simulink model "brain"  (Simulink 7.5)
settings: Solver=FixedStepDiscrete  StartTime=0.0  StopTime=inf  FixedStep=0.2  RelTol=1e-3
values from neighbouring files (symbols this model uses):
  Buoy1_Hue = 0.4    [brainconstants.m]    (also in brainconstants_David.m = 30)
  Buoy1_Saturation = 1.0    (= 1)    [brainconstants.m]    (also in brainconstants_David.m)
  Buoy1_Value = 0.45    [brainconstants.m]    (also in brainconstants_David.m)
  Buoy2_Hue = 0.0    (= 0)    [brainconstants.m]    (also in brainconstants_David.m = 80)
  Buoy2_Saturation = 1.0    (= 1)    [brainconstants.m]    (also in brainconstants_David.m)
  Buoy2_Value = 0.75    [brainconstants.m]    (also in brainconstants_David.m)
  Buoy_Max_Eccentricity = 0.7    [brainconstants.m]    (also in brainconstants_David.m = 1.2)
  Buoy_Max_Extent = 0.9    [brainconstants.m]    (also in brainconstants_David.m)
  Buoy_Min_Eccentricity = 0    [brainconstants.m]    (also in brainconstants_David.m)
  Buoy_Min_Extent = 0.7    [brainconstants.m]    (also in brainconstants_David.m = 0.1)
  Buoy_Strafe = 40    [brainconstants.m]    (also in brainconstants_David.m)
  Cam_Down_Strafe_XPos_Kd = 0.0    (= 0)    [brainconstants.m]    (also in brainconstants_David.m)
  Cam_Down_Strafe_XPos_Ki = 0.0    (= 0)    [brainconstants.m]    (also in brainconstants_David.m)
  Cam_Down_Strafe_XPos_Kp = -1.0    (= -1)    [brainconstants.m]    (also in brainconstants_David.m)
  Cam_Down_Yaw_XPos_Kd = 0.0    (= 0)    [brainconstants.m]    (also in brainconstants_David.m)
  Cam_Down_Yaw_XPos_Ki = 0.0    (= 0)    [brainconstants.m]    (also in brainconstants_David.m)
  Cam_Down_Yaw_XPos_Kp = 0.6    [brainconstants.m]    (also in brainconstants_David.m)
  Cam_Down_YPos_Kd = 0.0    (= 0)    [brainconstants.m]    (also in brainconstants_David.m)
  Cam_Down_YPos_Ki = 0.0    (= 0)    [brainconstants.m]    (also in brainconstants_David.m)
  Cam_Down_YPos_Kp = 0.75    [brainconstants.m]    (also in brainconstants_David.m)
  Cam_Forward_XPosition_Kd = 0.0    (= 0)    [brainconstants.m]    (also in brainconstants_David.m)
  Cam_Forward_XPosition_Ki = 0.0    (= 0)    [brainconstants.m]    (also in brainconstants_David.m)
  Cam_Forward_XPosition_Kp = 0.07    [brainconstants.m]    (also in brainconstants_David.m)
  Cam_Forward_YPosition_Kd = 0.0    (= 0)    [brainconstants.m]    (also in brainconstants_David.m)
  Cam_Forward_YPosition_Ki = 0.0    (= 0)    [brainconstants.m]    (also in brainconstants_David.m)
  Cam_Forward_YPosition_Kp = 0.8    [brainconstants.m]    (also in brainconstants_David.m)
  Depth_Kd = 0.0    (= 0)    [brainconstants.m]    (also in brainconstants_David.m)
  Depth_Ki = 0.0    (= 0)    [brainconstants.m]    (also in brainconstants_David.m)
  Depth_Kp = 75    [brainconstants.m]    (also in brainconstants_David.m)
  Heading_Forward_Velocity = 30    [brainconstants.m]    (also in brainconstants_David.m)
  Heading_Kd = 0.4    [brainconstants.m]    (also in brainconstants_David.m)
  Heading_Ki = 0.0    (= 0)    [brainconstants.m]    (also in brainconstants_David.m)
  Heading_Kp = 0.65    [brainconstants.m]    (also in brainconstants_David.m)
  Hedge_Hue = .4    (= 0.4)    [brainconstants.m]    (also in brainconstants_David.m)
  Hedge_Saturation = 1    [brainconstants.m]    (also in brainconstants_David.m)
  Hedge_Value = .75    (= 0.75)    [brainconstants.m]    (also in brainconstants_David.m)
  Iter_Segment_Thresh = 60    [brainconstants.m]    (also in brainconstants_David.m)
  MissionPlan = [1 1 1 1 1 1 1 1 1 1 1 1 1 0 0 0 0 0 0 0]    [brainconstants.m]    (also in brainconstants_David.m)
  Track_Desired_Depth = 8    [brainconstants.m]    (also in brainconstants_David.m)
  Track_HueHigher = 0.75    [brainconstants.m]    (also in brainconstants_David.m)
  Track_HueLower = 0.4    [brainconstants.m]    (also in brainconstants_David.m)
  Track_Min_Eccentricity = 0.9    [brainconstants.m]    (also in brainconstants_David.m)
  Track_Saturation = 0.75    [brainconstants.m]    (also in brainconstants_David.m)
  Vision_Forward_Velocity = 15    [brainconstants.m]    (also in brainconstants_David.m)
undefined symbols (not defined in the file or in its folder): DiscIntNeverNeededParam, gray, Rec, SDTV, strel, YawRate_Kd, YawRate_Ki, YawRate_Kp
libraries: vipconversions x32, simulink x26, vipgeotforms x9, vipstatistics x9, viptextngfix x7, vipmorphops x6, viptransforms x4, vipsnks x3, vipsrcs x1
(part 1 of 6)
settings Model: Creator=Stephen  LastModifiedBy=Stephen  ParamWorkspaceSource=ReferencedWorkspace  TunableVars=Buoy1_Hue,Buoy1_Saturation,Buoy1_Value,Buoy2_Hue,Buoy2_Saturation,Buoy2_Value,Buoy_Max_Eccentricity,Buoy_Max_Extent,Buoy_Min_Eccentricity,Buoy_Min_Extent,Buoy_Strafe,Cam_Down_Strafe_XPos_Kd,Cam_Down_Strafe_XPos_Ki,Cam_Down_Strafe_XPos_Kp,Cam_Down_XPos_Kd,Cam_Down_XPos_Ki,Cam_Down_XPos_Kp,Cam_Down_YPos_Kd,Cam_Down_YPos_Ki,Cam_Down_YPos_Kp,Cam_Down_Yaw_XPos_Kd,Cam_Down_Yaw_XPos_Ki,Cam_Down_Yaw_XPos_Kp,Cam_Forward_XPosition_Kd,Cam_Forward_XPosition_Ki,Cam_Forward_XPosition_Kp,Cam_Forward_YPosition_Kd,Cam_Forward_YPosition_Ki,Cam_Forward_YPosition_Kp,Depth_Kd,Depth_Ki,Depth_Kp,Heading_Forward_Velocity,Heading_Kd,Heading_Ki,Heading_Kp,Hedge_Hue,Hedge_Saturation,Hedge_Value,Iter_Segment_Thresh,Max_Blob_Size,Min_Blob_Size,MissionPlan,Track_Desired_Depth,Track_HueHigher,Track_HueLower,Track_Min_Eccentricity,Track_Saturation,Vision_Forward_Velocity  TunableVarsStorageClass=Auto,Auto,Auto,Auto,Auto,Auto,Auto,Auto,Auto,Auto,Auto,Auto,Auto,Auto,Auto,Auto,Auto,Auto,Auto,Auto,Auto,Auto,Auto,Auto,Auto,Auto,Auto,Auto,Auto,Auto,Auto,Auto,Auto,Auto,Auto,Auto,Auto,Auto,Auto,Auto,Auto,Auto,Auto,Auto,Auto,Auto,Auto,Auto,Auto  TunableVarsTypeQualifier=,,,,,,,,,,,,,,,,,,,,,,,,,,,,,,,,,,,,,,,,,,,,,,,,
settings DataIOCC: SaveFormat=Structure
settings OptimizationCC: InlineParams=on  OptimizeModelRefInitCode=on  LifeSpan=1
settings DebuggingCC: InheritedTsInSrcMsg=none  StrictBusMsg=Warning
settings HardwareCC: ProdIntDivRoundTo=Zero  ProdEndianess=LittleEndian  ProdHWDeviceType=AMD->K5/K6/Athlon
settings RTWCC: SystemTargetFile=ert.tlc  GenCodeOnly=on  GenerateMakefile=off  TemplateMakefile=ert_default_tmf  PostCodeGenCommand=packNGo(buildInfo);  Description=Real-Time Workshop Embedded Coder  RTWVerbose=off  ProcessScript=ert_make_rtw_hook  TargetLang=C++  RTWCompilerOptimization=On
settings CodeAppCC: IgnoreCustomStorageClasses=off  SimulinkDataObjDesc=on  SFDataObjDesc=on  InsertBlockDesc=on  ReqsInCode=on
settings ERTTargetCC: MultiwordLength=2048  IncludeMdlTerminateFcn=off  InlinedParameterPlacement=NonHierarchical  ERTCustomFileTemplate=example_file_process.tlc  ConvertIfToSwitch=off

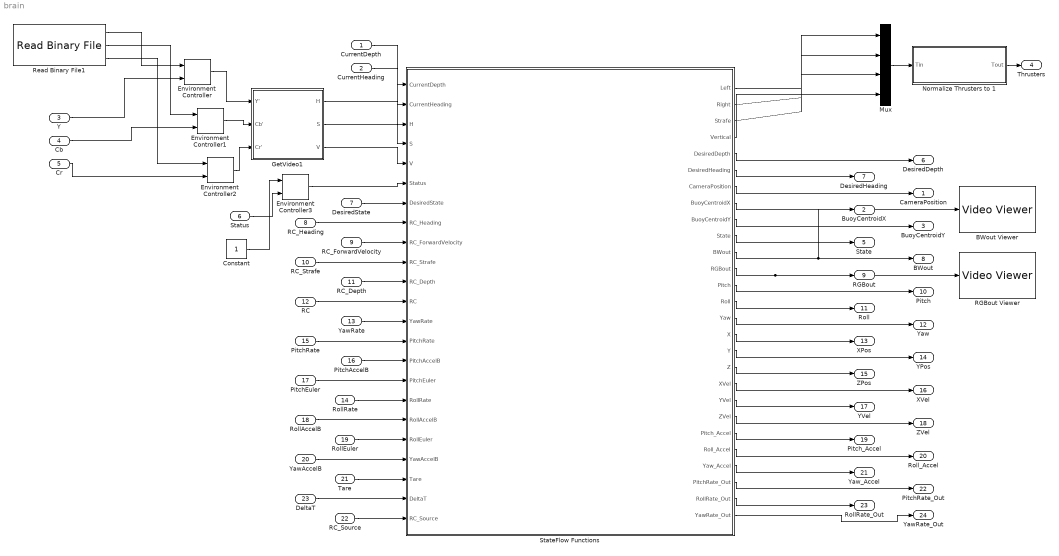
== system brain ==
  CurrentDepth : Inport  OutDataType=fixdt(1, 16)  OutScaling=2^0
  CurrentHeading : Inport  Port=2  OutDataType=fixdt(1, 16)  OutScaling=2^0
  Y : Inport  Port=3  PortDimensions=[480 640]  DataType=uint8  OutDataType=fixdt(1, 16)  OutScaling=2^0  OutDataTypeStr=uint8
  Cb : Inport  Port=4  PortDimensions=[240 320]  DataType=uint8  OutDataType=fixdt(1, 16)  OutScaling=2^0  OutDataTypeStr=uint8
  Cr : Inport  Port=5  PortDimensions=[240 320]  DataType=uint8  OutDataType=fixdt(1, 16)  OutScaling=2^0  OutDataTypeStr=uint8
  Status : Inport  Port=6  DataType=int8  OutDataType=fixdt(1, 16)  OutScaling=2^0  OutDataTypeStr=int8
  DesiredState : Inport  Port=7  OutDataType=fixdt(1, 16)  OutScaling=2^0
  RC_Heading : Inport  Port=8  OutDataType=fixdt(1, 16)  OutScaling=2^0
  RC_ForwardVelocity : Inport  Port=9  OutDataType=fixdt(1, 16)  OutScaling=2^0
  RC_Strafe : Inport  Port=10  OutDataType=fixdt(1, 16)  OutScaling=2^0
  RC_Depth : Inport  Port=11  OutDataType=fixdt(1, 16)  OutScaling=2^0
  RC : Inport  Port=12  OutDataType=fixdt(1, 16)  OutScaling=2^0
  YawRate : Inport  Port=13  OutDataType=fixdt(1, 16)  OutScaling=2^0
  RollRate : Inport  Port=14  OutDataType=fixdt(1, 16)  OutScaling=2^0
  PitchRate : Inport  Port=15  OutDataType=fixdt(1, 16)  OutScaling=2^0
  PitchAccelB : Inport  Port=16  OutDataType=fixdt(1, 16)  OutScaling=2^0
  PitchEuler : Inport  Port=17  OutDataType=fixdt(1, 16)  OutScaling=2^0
  RollAccelB : Inport  Port=18  OutDataType=fixdt(1, 16)  OutScaling=2^0
  RollEuler : Inport  Port=19  OutDataType=fixdt(1, 16)  OutScaling=2^0
  YawAccelB : Inport  Port=20  OutDataType=fixdt(1, 16)  OutScaling=2^0
  Tare : Inport  Port=21  OutDataType=fixdt(1, 16)  OutScaling=2^0
  RC_Source : Inport  Port=22  OutDataType=fixdt(1, 16)  OutScaling=2^0
  DeltaT : Inport  Port=23  OutDataType=fixdt(1, 16)  OutScaling=2^0
  BWout Viewer : vipsnks/Video Viewer  DialogControllerArgs=DataTag1  inputType=Obsolete7b  imagePorts=One multidimensional signal  useColorMap=off  colormapValue=gray(256)  specRange=off  minInputVal=0  maxInputVal=255  FigPos=[586 450 254 150]  AxisZoom=on  trueSizedOnce=off  OpenAtMdlStart=on
  Constant : Constant  OutDataTypeMode=int8  OutDataType=fixdt(1, 16)  OutScaling=2^0  OutDataTypeStr=int8
  Environment Controller{,1..3} (4 alike) : simulink/Signal Routing/Environment Controller  SystemSampleTime=-1
  GetVideo1 : Subsystem
  Mux : Mux
  Normalize Thrusters to 1 : Stateflow chart  TreatAsAtomicUnit=on
  RGBout Viewer : vipsnks/Video Viewer  DialogControllerArgs=DataTag8  inputType=Obsolete7b  imagePorts=One multidimensional signal  useColorMap=off  colormapValue=gray(256)  specRange=off  minInputVal=0  maxInputVal=255  FigPos=[469 292 254 150]  AxisZoom=on  trueSizedOnce=off  OpenAtMdlStart=on
  Read Binary File1 : vipsrcs/Read Binary File  DialogController=vipDDGCreate  DialogControllerArgs=DataTag9  FileName=vipmen.bin  loopOrNot=on  numLoops=1  VideoFormat=Four character codes  FOURCC=I420  BitStreamFormat=Planar  NumOutputs=3  ComponentOrder=[1 2 3]  Interlaced=off  LineOrdering=Top line first  Ts=-1  Component1=Y'  Component2=Cb  Component3=Cr  Component4=Alpha  Bits1=8  Bits2=8  Bits3=8  Bits4=8  Rows1=120  Rows2=60  Rows3=60  Rows4=288  Cols1=160  Cols2=80  Cols3=80  Cols4=352  YRows=480  YCols=640  SignedOutput=off  FileEndian=Little endian  OutputEOF=off
  StateFlow Functions : Stateflow chart  TreatAsAtomicUnit=on
  CameraPosition : Outport  OutDataType=fixdt(1, 16)  OutScaling=2^0
  BuoyCentroidX : Outport  Port=2  OutDataType=fixdt(1, 16)  OutScaling=2^0
  BuoyCentroidY : Outport  Port=3  OutDataType=fixdt(1, 16)  OutScaling=2^0
  Thrusters : Outport  Port=4  OutDataType=fixdt(1, 16)  OutScaling=2^0
  State : Outport  Port=5  OutDataType=fixdt(1, 16)  OutScaling=2^0
  DesiredDepth : Outport  Port=6  OutDataType=fixdt(1, 16)  OutScaling=2^0
  DesiredHeading : Outport  Port=7  OutDataType=fixdt(1, 16)  OutScaling=2^0
  BWout : Outport  Port=8  OutDataType=fixdt(1, 16)  OutScaling=2^0
  RGBout : Outport  Port=9  PortDimensions=[120 160 3]  OutDataType=fixdt(1, 16)  OutScaling=2^0
  Pitch : Outport  Port=10  OutDataType=fixdt(1, 16)  OutScaling=2^0
  Roll : Outport  Port=11  OutDataType=fixdt(1, 16)  OutScaling=2^0
  Yaw : Outport  Port=12  OutDataType=fixdt(1, 16)  OutScaling=2^0
  XPos : Outport  Port=13  OutDataType=fixdt(1, 16)  OutScaling=2^0
  YPos : Outport  Port=14  OutDataType=fixdt(1, 16)  OutScaling=2^0
  ZPos : Outport  Port=15  OutDataType=fixdt(1, 16)  OutScaling=2^0
  XVel : Outport  Port=16  OutDataType=fixdt(1, 16)  OutScaling=2^0
  YVel : Outport  Port=17  OutDataType=fixdt(1, 16)  OutScaling=2^0
  ZVel : Outport  Port=18  OutDataType=fixdt(1, 16)  OutScaling=2^0
  Pitch_Accel : Outport  Port=19  OutDataType=fixdt(1, 16)  OutScaling=2^0
  Roll_Accel : Outport  Port=20  OutDataType=fixdt(1, 16)  OutScaling=2^0
  Yaw_Accel : Outport  Port=21  OutDataType=fixdt(1, 16)  OutScaling=2^0
  PitchRate_Out : Outport  Port=22  OutDataType=fixdt(1, 16)  OutScaling=2^0
  RollRate_Out : Outport  Port=23  OutDataType=fixdt(1, 16)  OutScaling=2^0
  YawRate_Out : Outport  Port=24  OutDataType=fixdt(1, 16)  OutScaling=2^0
  wires:
  StateFlow Functions/7(CameraPosition) -> CameraPosition/1
  StateFlow Functions/8(BuoyCentroidX) -> BuoyCentroidX/1
  StateFlow Functions/9(BuoyCentroidY) -> BuoyCentroidY/1
  CurrentDepth/1 -> StateFlow Functions/1(CurrentDepth)
  CurrentHeading/1 -> StateFlow Functions/2(CurrentHeading)
  StateFlow Functions/10(State) -> State/1
  StateFlow Functions/5(DesiredDepth) -> DesiredDepth/1
  StateFlow Functions/6(DesiredHeading) -> DesiredHeading/1
  DesiredState/1 -> StateFlow Functions/7(DesiredState)
  RC_Heading/1 -> StateFlow Functions/8(RC_Heading)
  RC_ForwardVelocity/1 -> StateFlow Functions/9(RC_ForwardVelocity)
  RC_Strafe/1 -> StateFlow Functions/10(RC_Strafe)
  RC_Depth/1 -> StateFlow Functions/11(RC_Depth)
  RC/1 -> StateFlow Functions/12(RC)
  StateFlow Functions/2(Right) -> Mux/2
  StateFlow Functions/1(Left) -> Mux/1
  StateFlow Functions/3(Strafe) -> Mux/3
  StateFlow Functions/4(Vertical) -> Mux/4
  Status/1 -> Environment Controller3/2
  Environment Controller3/1 -> StateFlow Functions/6(Status)
  Constant/1 -> Environment Controller3/1
  StateFlow Functions/11(BWout) -> BWout/1, BWout Viewer/1
  Mux/1 -> Normalize Thrusters to 1/1(Tin)
  Normalize Thrusters to 1/1(Tout) -> Thrusters/1
  StateFlow Functions/12(RGBout) -> RGBout/1, RGBout Viewer/1
  GetVideo1/1(H) -> StateFlow Functions/3(H)
  GetVideo1/2(S) -> StateFlow Functions/4(S)
  GetVideo1/3(V) -> StateFlow Functions/5(V)
  Y/1 -> Environment Controller/2
  Cb/1 -> Environment Controller1/2
  Cr/1 -> Environment Controller2/2
  Environment Controller/1 -> GetVideo1/1(Y')
  Environment Controller1/1 -> GetVideo1/2(Cb')
  Environment Controller2/1 -> GetVideo1/3(Cr')
  Read Binary File1/1 -> Environment Controller/1
  Read Binary File1/2 -> Environment Controller1/1
  Read Binary File1/3 -> Environment Controller2/1
  YawRate/1 -> StateFlow Functions/13(YawRate)
  RollRate/1 -> StateFlow Functions/17(RollRate)
  PitchRate/1 -> StateFlow Functions/14(PitchRate)
  PitchAccelB/1 -> StateFlow Functions/15(PitchAccelB)
  PitchEuler/1 -> StateFlow Functions/16(PitchEuler)
  RollAccelB/1 -> StateFlow Functions/18(RollAccelB)
  RollEuler/1 -> StateFlow Functions/19(RollEuler)
  YawAccelB/1 -> StateFlow Functions/20(YawAccelB)
  Tare/1 -> StateFlow Functions/21(Tare)
  RC_Source/1 -> StateFlow Functions/23(RC_Source)
  StateFlow Functions/13(Pitch) -> Pitch/1
  StateFlow Functions/14(Roll) -> Roll/1
  StateFlow Functions/15(Yaw) -> Yaw/1
  StateFlow Functions/16(X) -> XPos/1
  StateFlow Functions/17(Y) -> YPos/1
  StateFlow Functions/18(Z) -> ZPos/1
  StateFlow Functions/19(XVel) -> XVel/1
  StateFlow Functions/20(YVel) -> YVel/1
  StateFlow Functions/21(ZVel) -> ZVel/1
  StateFlow Functions/22(Pitch_Accel) -> Pitch_Accel/1
  StateFlow Functions/23(Roll_Accel) -> Roll_Accel/1
  StateFlow Functions/24(Yaw_Accel) -> Yaw_Accel/1
  StateFlow Functions/25(PitchRate_Out) -> PitchRate_Out/1
  StateFlow Functions/26(RollRate_Out) -> RollRate_Out/1
  StateFlow Functions/27(YawRate_Out) -> YawRate_Out/1
  DeltaT/1 -> StateFlow Functions/22(DeltaT)

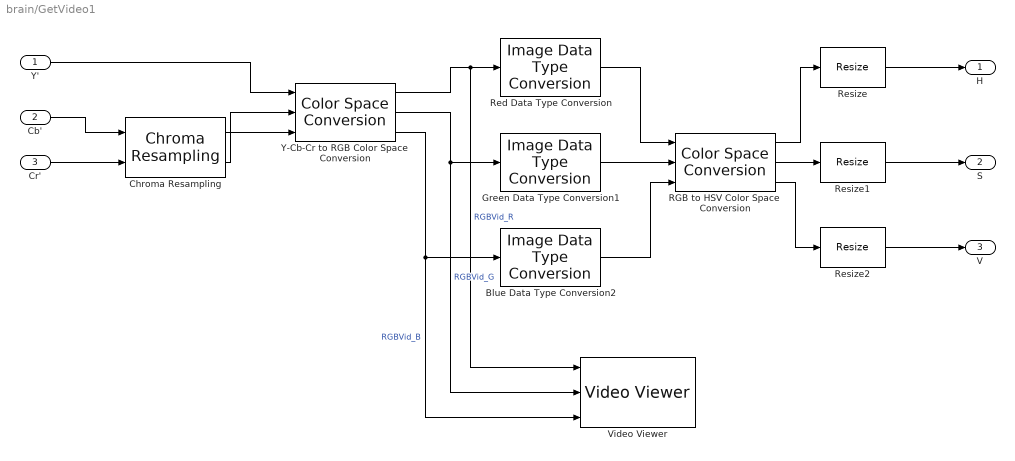
== system brain/GetVideo1 ==
  Y' : Inport  PortDimensions=[480 640]  OutDataType=fixdt(1, 16)  OutScaling=2^0
  Cb' : Inport  Port=2  PortDimensions=[240 320]  OutDataType=fixdt(1, 16)  OutScaling=2^0
  Cr' : Inport  Port=3  PortDimensions=[240 320]  OutDataType=fixdt(1, 16)  OutScaling=2^0
  Blue Data Type Conversion2 : vipconversions/Image Data Type Conversion  outDT=single  isSigned=on  wordLen=16  numFracBits=0
  Chroma Resampling : vipconversions/Chroma Resampling  resampling=4:2:0 (MPEG1) to 4:4:4  interpolation=pixel replication  antialiasing=Default  hcoeff=[0.2 0.6 0.2]  vcoeff=[0.5 0.5]  isInputTransposed=off
  Green Data Type Conversion1 : vipconversions/Image Data Type Conversion  outDT=single  isSigned=on  wordLen=16  numFracBits=0
  RGB to HSV Color Space  Conversion : vipconversions/Color Space  Conversion  conversion=Obsolete  conversionActive=R'G'B' to HSV  wp_str=D65  rec=Rec. 601 (SDTV)  sys=1125/60/2:1  imagePorts=Separate color signals
  Red Data Type Conversion : vipconversions/Image Data Type Conversion  outDT=single  isSigned=on  wordLen=16  numFracBits=0
  Resize : vipgeotforms/Resize  DialogController=vipDDGCreate  DialogControllerArgs=DataTag2  specify=Number of output rows and columns  rfactor=[200 150]  outCols=25  outRows=25  outRowsCols=[120 160]  interp_method=Bilinear  antialias=on  useROI=off  roiFlag=off  prodOutputMode=Binary point scaling  prodOutputWordLength=32  prodOutputFracLength=10  roundingMode=Nearest  overflowMode=on
  Resize1 : vipgeotforms/Resize  DialogController=vipDDGCreate  DialogControllerArgs=DataTag3  specify=Number of output rows and columns  rfactor=[200 150]  outCols=25  outRows=25  outRowsCols=[120 160]  interp_method=Bilinear  antialias=on  useROI=off  roiFlag=off  prodOutputMode=Binary point scaling  prodOutputWordLength=32  prodOutputFracLength=10  roundingMode=Nearest  overflowMode=on
  Resize2 : vipgeotforms/Resize  DialogController=vipDDGCreate  DialogControllerArgs=DataTag4  specify=Number of output rows and columns  rfactor=[200 150]  outCols=25  outRows=25  outRowsCols=[120 160]  interp_method=Bilinear  antialias=on  useROI=off  roiFlag=off  prodOutputMode=Binary point scaling  prodOutputWordLength=32  prodOutputFracLength=10  roundingMode=Nearest  overflowMode=on
  Video Viewer : vipsnks/Video Viewer  DialogControllerArgs=DataTag6  inputType=Obsolete7b  imagePorts=Separate color signals  useColorMap=off  colormapValue=gray(256)  specRange=off  minInputVal=0  maxInputVal=255  FigPos=[307 461 590 252]  AxisZoom=on  trueSizedOnce=off  OpenAtMdlStart=on
  Y-Cb-Cr to RGB Color Space  Conversion : vipconversions/Color Space  Conversion  conversion=Obsolete  conversionActive=Y'CbCr to R'G'B'  wp_str=D65  rec=Rec. 601 (SDTV)  sys=1125/60/2:1  imagePorts=Separate color signals
  H : Outport
  S : Outport  Port=2
  V : Outport  Port=3
  wires:
  RGB to HSV Color Space  Conversion/3 -> Resize2/1
  RGB to HSV Color Space  Conversion/2 -> Resize1/1
  RGB to HSV Color Space  Conversion/1 -> Resize/1
  Blue Data Type Conversion2/1 -> RGB to HSV Color Space  Conversion/3
  Green Data Type Conversion1/1 -> RGB to HSV Color Space  Conversion/2
  Red Data Type Conversion/1 -> RGB to HSV Color Space  Conversion/1
  Y-Cb-Cr to RGB Color Space  Conversion/3 -> Blue Data Type Conversion2/1, Video Viewer/3  "RGBVid_B"
  Y-Cb-Cr to RGB Color Space  Conversion/2 -> Green Data Type Conversion1/1, Video Viewer/2  "RGBVid_G"
  Y-Cb-Cr to RGB Color Space  Conversion/1 -> Red Data Type Conversion/1, Video Viewer/1  "RGBVid_R"
  Chroma Resampling/2 -> Y-Cb-Cr to RGB Color Space  Conversion/3
  Chroma Resampling/1 -> Y-Cb-Cr to RGB Color Space  Conversion/2
  Resize/1 -> H/1
  Resize1/1 -> S/1
  Resize2/1 -> V/1
  Y'/1 -> Y-Cb-Cr to RGB Color Space  Conversion/1
  Cb'/1 -> Chroma Resampling/1
  Cr'/1 -> Chroma Resampling/2

== system brain/StateFlow Functions/StateFlowFunctions.Buoys.ApproachBuoys.ApproachFirstBuoy.GetFirstBuoyStats ==
  f : TriggerPort  TriggerType=function-call
      settings: CopyFcn=set_param(gcbh,'PreDeleteFcn','')  PreDeleteFcn=Stateflow.SLINSF.SimulinkMan.unsafePredeleteFcn
  Constant : Constant  Value=Buoy1_Hue  OutDataType=fixdt(1, 16)  OutScaling=2^0  SampleTime=-1
  Constant1 : Constant  Value=Buoy1_Value  OutDataType=fixdt(1, 16)  OutScaling=2^0  SampleTime=-1
  Constant2 : Constant  Value=Buoy1_Saturation  OutDataType=fixdt(1, 16)  OutScaling=2^0  SampleTime=-1
  B_H : Outport
  B_S : Outport  Port=2
  B_V : Outport  Port=3
  wires:
  Constant/1 -> B_H/1
  Constant2/1 -> B_S/1
  Constant1/1 -> B_V/1

== system brain/StateFlow Functions/StateFlowFunctions.Buoys.ApproachBuoys.ApproachFirstBuoy.WhichBuoysToApproach ==
  note: FirstD and SecondD can be 1,2,3 corresponding to left, middle or right
  buoys : Inport  PortDimensions=[50 4]
  num_blobs : Inport  Port=2
  f : TriggerPort  TriggerType=function-call
      settings: CopyFcn=set_param(gcbh,'PreDeleteFcn','')  PreDeleteFcn=Stateflow.SLINSF.SimulinkMan.unsafePredeleteFcn
  FirstBuoy Info : Subsystem
  GetBestColorMatch : Stateflow chart  TreatAsAtomicUnit=on
  Second Buoy Info : Subsystem
  FirstD : Outport
  SecondD : Outport  Port=2
  wires:
  buoys/1 -> GetBestColorMatch/1(Buoys)
  num_blobs/1 -> GetBestColorMatch/8(num_blobs)
  FirstBuoy Info/1(Out1) -> GetBestColorMatch/2(B1_L)
  FirstBuoy Info/2(Out2) -> GetBestColorMatch/3(B1_a)
  FirstBuoy Info/3(Out3) -> GetBestColorMatch/4(B1_b)
  Second Buoy Info/1(Out1) -> GetBestColorMatch/5(B2_L)
  Second Buoy Info/2(Out2) -> GetBestColorMatch/6(B2_a)
  Second Buoy Info/3(Out3) -> GetBestColorMatch/7(B2_b)
  GetBestColorMatch/1(Direction1) -> FirstD/1
  GetBestColorMatch/2(Direction2) -> SecondD/1

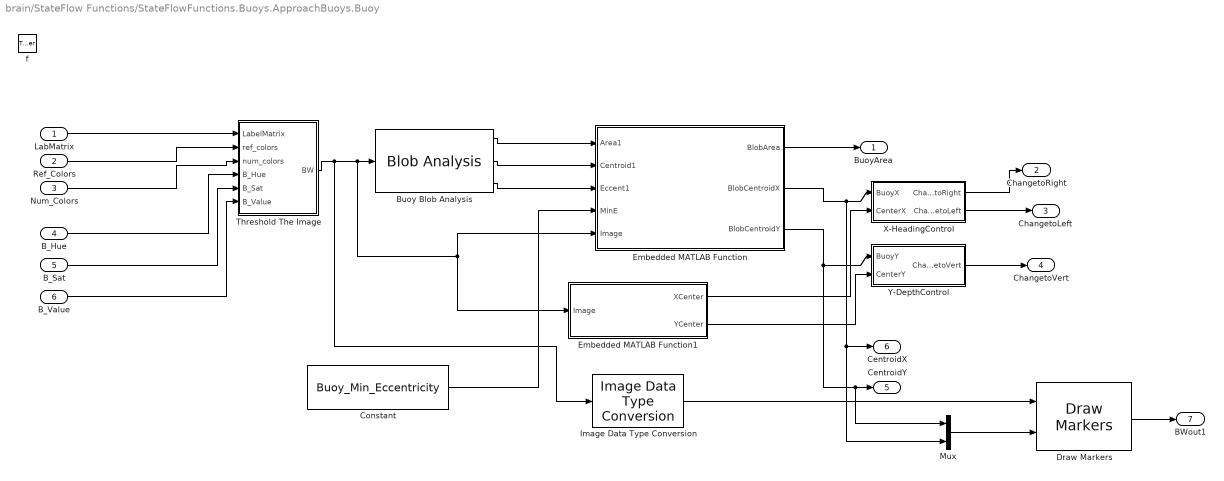
== system brain/StateFlow Functions/StateFlowFunctions.Buoys.ApproachBuoys.Buoy ==
  LabMatrix : Inport  PortDimensions=[120 160]
  Ref_Colors : Inport  Port=2  PortDimensions=[50 3]
  Num_Colors : Inport  Port=3  PortDimensions=1
  B_Hue : Inport  Port=4
  B_Sat : Inport  Port=5
  B_Value : Inport  Port=6
  f : TriggerPort  TriggerType=function-call
      settings: CopyFcn=set_param(gcbh,'PreDeleteFcn','')  PreDeleteFcn=Stateflow.SLINSF.SimulinkMan.unsafePredeleteFcn
  Buoy Blob Analysis : vipstatistics/Blob Analysis  Tag=vipblks_row_conv  DialogController=vipDDGCreate  DialogControllerArgs=DataTag10  area=on  centroid=on  bBox=off  majorAxis=off  minorAxis=off  angle=off  eccentricity=on  equivDiameterSq=off  extent=off  perimeter=off  maxBlobs=Max_Num_Blobs_Buoy  warnIfNumBlobsExceeded=off  isCount=off  useMinArea=on  minArea=Min_Blob_Size  useMaxArea=on  maxArea=Max_Blob_Size  excludeBorderBlob=off  outDT=double  isOutVarDim=off  isFill=on  fillValues=-1  conn=8  isLabel=off  outputMode=Binary point scaling  outputWordLength=32  outputFracLength=16  firstCoeffMode=Binary point scaling  firstCoeffWordLength=16  firstCoeffFracLength=14  secondCoeffMode=Binary point scaling  secondCoeffWordLength=32  secondCoeffFracLength=16  accumMode=Binary point scaling  accumWordLength=32  accumFracLength=0  prodOutputMode=Binary point scaling  prodOutputWordLength=32  prodOutputFracLength=16  roundingMode=Floor  overflowMode=off
  Constant : Constant  Value=Buoy_Min_Eccentricity  OutDataType=fixdt(1, 16)  OutScaling=2^0  SampleTime=-1
  Draw Markers : viptextngfix/Draw Markers  DialogController=vipDDGCreate  DialogControllerArgs=DataTag11  shape=X-mark  size=7  fill=off  fillClrSource=Specify via dialog  display=User-specified value  intensity=200  color=.5  opacity=0.6  viewport=Entire image  antialiasing=off  inType=Obsolete  imagePorts=One multidimensional signal  prodOutputMode=Binary point scaling  prodOutputWordLength=32  prodOutputFracLength=14  memoryMode=Specify word length  memoryWordLength=16  memoryFracLength=15  roundingMode=Floor  overflowMode=off
  Embedded MATLAB Function : Stateflow chart  TreatAsAtomicUnit=on
  Embedded MATLAB Function1 : Stateflow chart  TreatAsAtomicUnit=on
  Image Data Type Conversion : vipconversions/Image Data Type Conversion  outDT=double  isSigned=on  wordLen=16  numFracBits=0
  Mux : Mux  Inputs=2
  Threshold The Image : Subsystem
  X-HeadingControl : Subsystem
  Y-DepthControl : Subsystem
  BuoyArea : Outport  OutDataType=fixdt(1, 16)  OutScaling=2^0
  ChangetoRight : Outport  Port=2  OutDataType=fixdt(1, 16)  OutScaling=2^0
  ChangetoLeft : Outport  Port=3  OutDataType=fixdt(1, 16)  OutScaling=2^0
  ChangetoVert : Outport  Port=4  OutDataType=fixdt(1, 16)  OutScaling=2^0
  CentroidY : Outport  Port=5  OutDataType=fixdt(1, 16)  OutScaling=2^0
  CentroidX : Outport  Port=6  OutDataType=fixdt(1, 16)  OutScaling=2^0
  BWout1 : Outport  Port=7  OutDataType=fixdt(1, 16)  OutScaling=2^0
  wires:
  X-HeadingControl/1(ChangetoRight) -> ChangetoRight/1
  X-HeadingControl/2(ChangetoLeft) -> ChangetoLeft/1
  Y-DepthControl/1(ChangetoVert) -> ChangetoVert/1
  Embedded MATLAB Function/1(BlobArea) -> BuoyArea/1
  Embedded MATLAB Function/2(BlobCentroidX) -> X-HeadingControl/1(BuoyX), CentroidX/1, Mux/2
  Embedded MATLAB Function/3(BlobCentroidY) -> Y-DepthControl/1(BuoyY), CentroidY/1, Mux/1
  Threshold The Image/1(BW) -> Image Data Type Conversion/1, Buoy Blob Analysis/1, Embedded MATLAB Function/5(Image), Embedded MATLAB Function1/1(Image)
  Embedded MATLAB Function1/1(XCenter) -> X-HeadingControl/2(CenterX)
  Embedded MATLAB Function1/2(YCenter) -> Y-DepthControl/2(CenterY)
  LabMatrix/1 -> Threshold The Image/1(LabelMatrix)
  Ref_Colors/1 -> Threshold The Image/2(ref_colors)
  Num_Colors/1 -> Threshold The Image/3(num_colors)
  Buoy Blob Analysis/1 -> Embedded MATLAB Function/1(Area1)
  Buoy Blob Analysis/2 -> Embedded MATLAB Function/2(Centroid1)
  Buoy Blob Analysis/3 -> Embedded MATLAB Function/3(Eccent1)
  Constant/1 -> Embedded MATLAB Function/4(MinE)
  B_Hue/1 -> Threshold The Image/4(B_Hue)
  B_Sat/1 -> Threshold The Image/5(B_Sat)
  B_Value/1 -> Threshold The Image/6(B_Value)
  Mux/1 -> Draw Markers/2
  Image Data Type Conversion/1 -> Draw Markers/1
  Draw Markers/1 -> BWout1/1

== system brain/StateFlow Functions/StateFlowFunctions.Buoys.ApproachBuoys.FindSecondBuoy.GetSecondBuoyStats ==
  f : TriggerPort  TriggerType=function-call
      settings: CopyFcn=set_param(gcbh,'PreDeleteFcn','')  PreDeleteFcn=Stateflow.SLINSF.SimulinkMan.unsafePredeleteFcn
  Constant : Constant  Value=Buoy2_Hue  OutDataType=fixdt(1, 16)  OutScaling=2^0  SampleTime=-1
  Constant1 : Constant  Value=Buoy2_Value  OutDataType=fixdt(1, 16)  OutScaling=2^0  SampleTime=-1
  Constant2 : Constant  Value=Buoy2_Saturation  OutDataType=fixdt(1, 16)  OutScaling=2^0  SampleTime=-1
  B_H : Outport
  B_S : Outport  Port=2
  B_V : Outport  Port=3
  wires:
  Constant/1 -> B_H/1
  Constant2/1 -> B_S/1
  Constant1/1 -> B_V/1

== system brain/StateFlow Functions/StateFlowFunctions.Buoys.ApproachBuoys.FindSecondBuoy.GetStrafe ==
  f : TriggerPort  TriggerType=function-call
      settings: CopyFcn=set_param(gcbh,'PreDeleteFcn','')  PreDeleteFcn=Stateflow.SLINSF.SimulinkMan.unsafePredeleteFcn
  Constant : Constant  Value=Buoy_Strafe  OutDataType=fixdt(1, 16)  OutScaling=2^0  SampleTime=-1
  Strafe1 : Outport
  wires:
  Constant/1 -> Strafe1/1

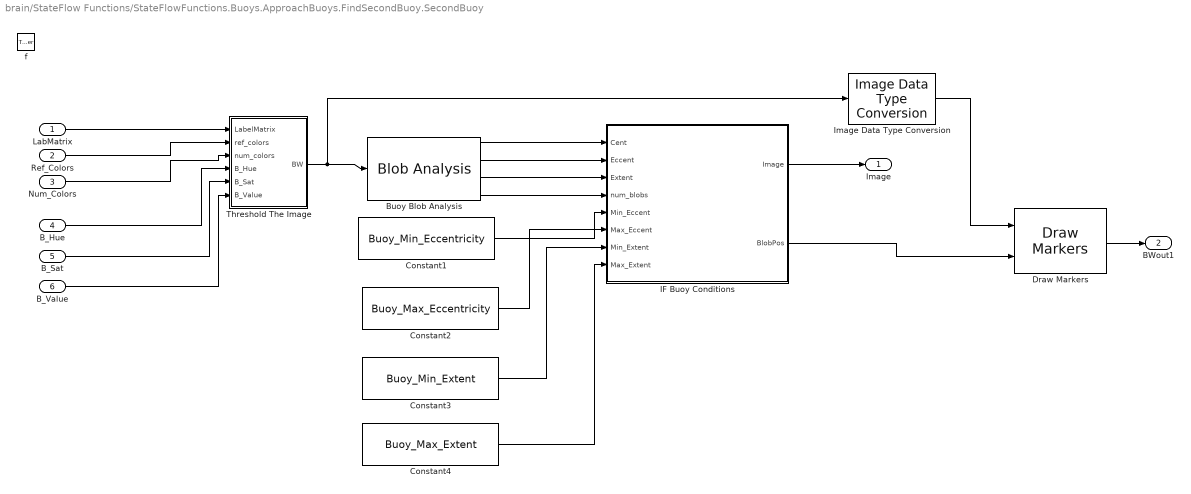
== system brain/StateFlow Functions/StateFlowFunctions.Buoys.ApproachBuoys.FindSecondBuoy.SecondBuoy ==
  LabMatrix : Inport  PortDimensions=[120 160]
  Ref_Colors : Inport  Port=2  PortDimensions=[50 3]
  Num_Colors : Inport  Port=3  PortDimensions=1
  B_Hue : Inport  Port=4
  B_Sat : Inport  Port=5
  B_Value : Inport  Port=6
  f : TriggerPort  TriggerType=function-call
      settings: CopyFcn=set_param(gcbh,'PreDeleteFcn','')  PreDeleteFcn=Stateflow.SLINSF.SimulinkMan.unsafePredeleteFcn
  Buoy Blob Analysis : vipstatistics/Blob Analysis  Tag=vipblks_row_conv  DialogController=vipDDGCreate  DialogControllerArgs=DataTag12  area=off  centroid=on  bBox=off  majorAxis=off  minorAxis=off  angle=off  eccentricity=on  equivDiameterSq=off  extent=on  perimeter=off  maxBlobs=Max_Num_Blobs_Buoy  warnIfNumBlobsExceeded=off  isCount=on  useMinArea=on  minArea=Min_Blob_Size  useMaxArea=on  maxArea=Max_Blob_Size  excludeBorderBlob=off  outDT=double  isOutVarDim=off  isFill=on  fillValues=-1  conn=8  isLabel=off  outputMode=Binary point scaling  outputWordLength=32  outputFracLength=16  firstCoeffMode=Binary point scaling  firstCoeffWordLength=16  firstCoeffFracLength=14  secondCoeffMode=Binary point scaling  secondCoeffWordLength=32  secondCoeffFracLength=16  accumMode=Binary point scaling  accumWordLength=32  accumFracLength=0  prodOutputMode=Binary point scaling  prodOutputWordLength=32  prodOutputFracLength=16  roundingMode=Floor  overflowMode=off
  Constant1 : Constant  Value=Buoy_Min_Eccentricity  OutDataType=fixdt(1, 16)  OutScaling=2^0  SampleTime=-1
  Constant2 : Constant  Value=Buoy_Max_Eccentricity  OutDataType=fixdt(1, 16)  OutScaling=2^0  SampleTime=-1
  Constant3 : Constant  Value=Buoy_Min_Extent  OutDataType=fixdt(1, 16)  OutScaling=2^0  SampleTime=-1
  Constant4 : Constant  Value=Buoy_Max_Extent  OutDataType=fixdt(1, 16)  OutScaling=2^0  SampleTime=-1
  Draw Markers : viptextngfix/Draw Markers  DialogController=vipDDGCreate  DialogControllerArgs=DataTag13  shape=X-mark  size=7  fill=off  fillClrSource=Specify via dialog  display=User-specified value  intensity=200  color=.75  opacity=0.6  viewport=Entire image  antialiasing=off  inType=Obsolete  imagePorts=One multidimensional signal  prodOutputMode=Binary point scaling  prodOutputWordLength=32  prodOutputFracLength=14  memoryMode=Specify word length  memoryWordLength=16  memoryFracLength=15  roundingMode=Floor  overflowMode=off
  IF Buoy Conditions : Stateflow chart  TreatAsAtomicUnit=on
  Image Data Type Conversion : vipconversions/Image Data Type Conversion  outDT=double  isSigned=on  wordLen=16  numFracBits=0
  Threshold The Image : Subsystem
  Image : Outport  OutDataType=fixdt(1, 16)  OutScaling=2^0
  BWout1 : Outport  Port=2  OutDataType=fixdt(1, 16)  OutScaling=2^0
  wires:
  Threshold The Image/1(BW) -> Buoy Blob Analysis/1, Image Data Type Conversion/1
  LabMatrix/1 -> Threshold The Image/1(LabelMatrix)
  Ref_Colors/1 -> Threshold The Image/2(ref_colors)
  Num_Colors/1 -> Threshold The Image/3(num_colors)
  B_Hue/1 -> Threshold The Image/4(B_Hue)
  B_Sat/1 -> Threshold The Image/5(B_Sat)
  B_Value/1 -> Threshold The Image/6(B_Value)
  Constant1/1 -> IF Buoy Conditions/5(Min_Eccent)
  Constant2/1 -> IF Buoy Conditions/6(Max_Eccent)
  Constant3/1 -> IF Buoy Conditions/7(Min_Extent)
  Constant4/1 -> IF Buoy Conditions/8(Max_Extent)
  IF Buoy Conditions/1(Image) -> Image/1
  Buoy Blob Analysis/1 -> IF Buoy Conditions/1(Cent)
  Buoy Blob Analysis/2 -> IF Buoy Conditions/2(Eccent)
  Buoy Blob Analysis/3 -> IF Buoy Conditions/3(Extent)
  Buoy Blob Analysis/4 -> IF Buoy Conditions/4(num_blobs)
  Image Data Type Conversion/1 -> Draw Markers/1
  IF Buoy Conditions/2(BlobPos) -> Draw Markers/2
  Draw Markers/1 -> BWout1/1

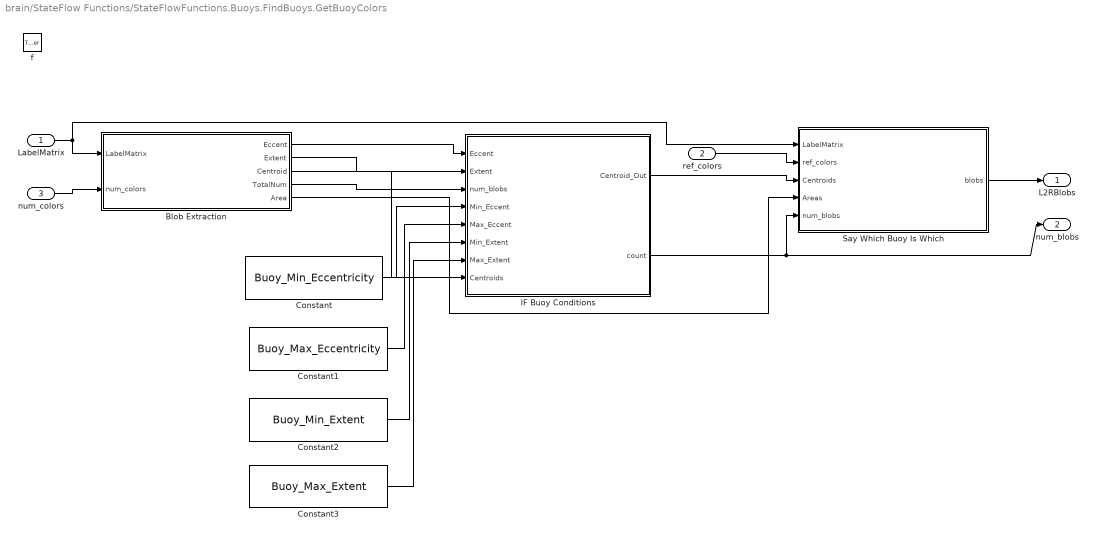
== system brain/StateFlow Functions/StateFlowFunctions.Buoys.FindBuoys.GetBuoyColors ==
  LabelMatrix : Inport  PortDimensions=[120 160]
  ref_colors : Inport  Port=2  PortDimensions=[50 ,3]
  num_colors : Inport  Port=3
  f : TriggerPort  TriggerType=function-call
      settings: CopyFcn=set_param(gcbh,'PreDeleteFcn','')  PreDeleteFcn=Stateflow.SLINSF.SimulinkMan.unsafePredeleteFcn
  Blob Extraction : Stateflow chart  TreatAsAtomicUnit=on
  Constant : Constant  Value=Buoy_Min_Eccentricity  OutDataType=fixdt(1, 16)  OutScaling=2^0  SampleTime=-1
  Constant1 : Constant  Value=Buoy_Max_Eccentricity  OutDataType=fixdt(1, 16)  OutScaling=2^0  SampleTime=-1
  Constant2 : Constant  Value=Buoy_Min_Extent  OutDataType=fixdt(1, 16)  OutScaling=2^0  SampleTime=-1
  Constant3 : Constant  Value=Buoy_Max_Extent  OutDataType=fixdt(1, 16)  OutScaling=2^0  SampleTime=-1
  IF Buoy Conditions : Stateflow chart  TreatAsAtomicUnit=on
  Say Which Buoy Is Which : Stateflow chart  TreatAsAtomicUnit=on
  L2RBlobs : Outport  PortDimensions=[50 4]
  num_blobs : Outport  Port=2
  wires:
  LabelMatrix/1 -> Blob Extraction/1(LabelMatrix), Say Which Buoy Is Which/1(LabelMatrix)
  num_colors/1 -> Blob Extraction/2(num_colors)
  Blob Extraction/1(Eccent) -> IF Buoy Conditions/1(Eccent)
  Blob Extraction/2(Extent) -> IF Buoy Conditions/2(Extent)
  Blob Extraction/4(TotalNum) -> IF Buoy Conditions/3(num_blobs)
  Constant/1 -> IF Buoy Conditions/4(Min_Eccent)
  Constant1/1 -> IF Buoy Conditions/5(Max_Eccent)
  Constant2/1 -> IF Buoy Conditions/6(Min_Extent)
  Constant3/1 -> IF Buoy Conditions/7(Max_Extent)
  Blob Extraction/3(Centroid) -> IF Buoy Conditions/8(Centroids)
  IF Buoy Conditions/1(Centroid_Out) -> Say Which Buoy Is Which/3(Centroids)
  ref_colors/1 -> Say Which Buoy Is Which/2(ref_colors)
  Say Which Buoy Is Which/1(blobs) -> L2RBlobs/1
  Blob Extraction/5(Area) -> Say Which Buoy Is Which/4(Areas)
  IF Buoy Conditions/2(count) -> Say Which Buoy Is Which/5(num_blobs), num_blobs/1

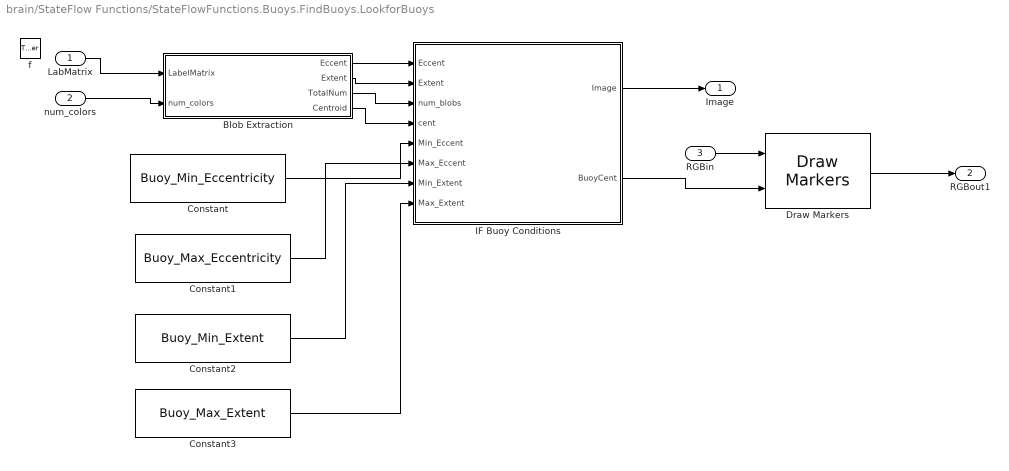
== system brain/StateFlow Functions/StateFlowFunctions.Buoys.FindBuoys.LookforBuoys ==
  LabMatrix : Inport  PortDimensions=[120 160]  OutDataType=fixdt(1, 16)  OutScaling=2^0
  num_colors : Inport  Port=2  OutDataType=fixdt(1, 16)  OutScaling=2^0
  RGBin : Inport  Port=3  PortDimensions=[120 160 3]  OutDataType=fixdt(1, 16)  OutScaling=2^0
  f : TriggerPort  TriggerType=function-call
      settings: CopyFcn=set_param(gcbh,'PreDeleteFcn','')  PreDeleteFcn=Stateflow.SLINSF.SimulinkMan.unsafePredeleteFcn
  Blob Extraction : Stateflow chart  TreatAsAtomicUnit=on
  Constant : Constant  Value=Buoy_Min_Eccentricity  OutDataType=fixdt(1, 16)  OutScaling=2^0  SampleTime=-1
  Constant1 : Constant  Value=Buoy_Max_Eccentricity  OutDataType=fixdt(1, 16)  OutScaling=2^0  SampleTime=-1
  Constant2 : Constant  Value=Buoy_Min_Extent  OutDataType=fixdt(1, 16)  OutScaling=2^0  SampleTime=-1
  Constant3 : Constant  Value=Buoy_Max_Extent  OutDataType=fixdt(1, 16)  OutScaling=2^0  SampleTime=-1
  Draw Markers : viptextngfix/Draw Markers  DialogController=vipDDGCreate  DialogControllerArgs=DataTag14  shape=X-mark  size=7  fill=off  fillClrSource=Specify via dialog  display=User-specified value  intensity=200  color=[0 0 0]  opacity=0.6  viewport=Entire image  antialiasing=off  inType=Obsolete  imagePorts=One multidimensional signal  prodOutputMode=Binary point scaling  prodOutputWordLength=32  prodOutputFracLength=14  memoryMode=Specify word length  memoryWordLength=16  memoryFracLength=15  roundingMode=Floor  overflowMode=off
  IF Buoy Conditions : Stateflow chart  TreatAsAtomicUnit=on
  Image : Outport  OutDataType=fixdt(1, 16)  OutScaling=2^0
  RGBout1 : Outport  Port=2  PortDimensions=[120 160 3]  OutDataType=fixdt(1, 16)  OutScaling=2^0
  wires:
  LabMatrix/1 -> Blob Extraction/1(LabelMatrix)
  num_colors/1 -> Blob Extraction/2(num_colors)
  Blob Extraction/1(Eccent) -> IF Buoy Conditions/1(Eccent)
  Blob Extraction/2(Extent) -> IF Buoy Conditions/2(Extent)
  Constant/1 -> IF Buoy Conditions/5(Min_Eccent)
  Constant1/1 -> IF Buoy Conditions/6(Max_Eccent)
  Constant2/1 -> IF Buoy Conditions/7(Min_Extent)
  Constant3/1 -> IF Buoy Conditions/8(Max_Extent)
  IF Buoy Conditions/1(Image) -> Image/1
  Blob Extraction/3(TotalNum) -> IF Buoy Conditions/3(num_blobs)
  Blob Extraction/4(Centroid) -> IF Buoy Conditions/4(cent)
  IF Buoy Conditions/2(BuoyCent) -> Draw Markers/2
  RGBin/1 -> Draw Markers/1
  Draw Markers/1 -> RGBout1/1

== system brain/StateFlow Functions/StateFlowFunctions.Buoys.GetBuoyForwardVelocity ==
  f : TriggerPort  TriggerType=function-call
      settings: CopyFcn=set_param(gcbh,'PreDeleteFcn','')  PreDeleteFcn=Stateflow.SLINSF.SimulinkMan.unsafePredeleteFcn
  Constant : Constant  Value=Heading_Forward_Velocity  OutDataType=fixdt(1, 16)  OutScaling=2^0  SampleTime=-1
  ForwardVel : Outport
  wires:
  Constant/1 -> ForwardVel/1

== system brain/StateFlow Functions/StateFlowFunctions.Buoys.IterativeSegmentation ==
  H : Inport  PortDimensions=[120 160]
  S : Inport  Port=2  PortDimensions=[120 160]
  V : Inport  Port=3  PortDimensions=[120 160]
  f : TriggerPort  TriggerType=function-call
      settings: CopyFcn=set_param(gcbh,'PreDeleteFcn','')  PreDeleteFcn=Stateflow.SLINSF.SimulinkMan.unsafePredeleteFcn
  Color Space  Conversion : vipconversions/Color Space  Conversion  conversion=Obsolete  conversionActive=HSV to R'G'B'  wp_str=D50  rec=Rec. 601 (SDTV)  sys=1125/60/2:1  imagePorts=Separate color signals
  Color Space  Conversion1 : vipconversions/Color Space  Conversion  conversion=Obsolete  conversionActive=sR'G'B' to L*a*b*  wp_str=D50  rec=Rec. 601 (SDTV)  sys=1125/60/2:1  imagePorts=Separate color signals
  Low Pass Filter : Subsystem
  Segmentation : Subsystem
  LabelMatrix : Outport  PortDimensions=[120 160]
  num_colors : Outport  Port=2
  Ref_Colors : Outport  Port=3
  wires:
  Color Space  Conversion/1 -> Low Pass Filter/1(R)
  Color Space  Conversion/2 -> Low Pass Filter/2(G)
  Color Space  Conversion/3 -> Low Pass Filter/3(B)
  Color Space  Conversion1/1 -> Segmentation/1(L)
  Color Space  Conversion1/2 -> Segmentation/2(a)
  Color Space  Conversion1/3 -> Segmentation/3(b)
  Low Pass Filter/1(R') -> Color Space  Conversion1/1
  Low Pass Filter/2(G') -> Color Space  Conversion1/2
  Low Pass Filter/3(B') -> Color Space  Conversion1/3
  H/1 -> Color Space  Conversion/1
  S/1 -> Color Space  Conversion/2
  V/1 -> Color Space  Conversion/3
  Segmentation/1(LabelMatrix) -> LabelMatrix/1
  Segmentation/2(num_colors) -> num_colors/1
  Segmentation/3(ref_colors) -> Ref_Colors/1

== system brain/StateFlow Functions/StateFlowFunctions.Buoys.ShowSegmentedImage ==
  LabMatrix : Inport  PortDimensions=[120 160]
  Ref_Colors : Inport  Port=2  PortDimensions=[50 3]
  f : TriggerPort  TriggerType=function-call
      settings: CopyFcn=set_param(gcbh,'PreDeleteFcn','')  PreDeleteFcn=Stateflow.SLINSF.SimulinkMan.unsafePredeleteFcn
  Color Space  Conversion : vipconversions/Color Space  Conversion  conversion=Obsolete  conversionActive=L*a*b* to sR'G'B'  wp_str=D50  rec=Rec. 601 (SDTV)  sys=1125/60/2:1  imagePorts=Separate color signals
  Embedded MATLAB Function : Stateflow chart  TreatAsAtomicUnit=on
  Embedded MATLAB Function1 : Stateflow chart  TreatAsAtomicUnit=on
  RGBout : Outport  PortDimensions=[120 160 3]  OutDataType=fixdt(1, 16)  OutScaling=2^0
  wires:
  LabMatrix/1 -> Embedded MATLAB Function/1(LabMatrix)
  Ref_Colors/1 -> Embedded MATLAB Function/2(Ref_Colors)
  Embedded MATLAB Function/1(L) -> Color Space  Conversion/1
  Embedded MATLAB Function/2(a) -> Color Space  Conversion/2
  Embedded MATLAB Function/3(b) -> Color Space  Conversion/3
  Color Space  Conversion/1 -> Embedded MATLAB Function1/1(R)
  Color Space  Conversion/2 -> Embedded MATLAB Function1/2(G)
  Color Space  Conversion/3 -> Embedded MATLAB Function1/3(B)
  Embedded MATLAB Function1/1(RGB) -> RGBout/1

== system brain/StateFlow Functions/StateFlowFunctions.FollowOnePath.MakeHSVImage ==
  H1 : Inport  PortDimensions=[120 160]
  S1 : Inport  Port=2  PortDimensions=[120 160]
  V1 : Inport  Port=3  PortDimensions=[120 160]
  f : TriggerPort  TriggerType=function-call
      settings: CopyFcn=set_param(gcbh,'PreDeleteFcn','')  PreDeleteFcn=Stateflow.SLINSF.SimulinkMan.unsafePredeleteFcn
  PutHSVImageTogether : Stateflow chart  TreatAsAtomicUnit=on
  HSVImage1 : Outport  PortDimensions=[120 160 3]
  wires:
  PutHSVImageTogether/1(HSVImage1) -> HSVImage1/1
  H1/1 -> PutHSVImageTogether/1(H)
  S1/1 -> PutHSVImageTogether/2(S)
  V1/1 -> PutHSVImageTogether/3(V)

== system brain/StateFlow Functions/StateFlowFunctions.FollowOnePath.OnePath.AlignWithPath.Align ==
  note: Error
  HeadingAlong : Inport
  f : TriggerPort  TriggerType=function-call
      settings: CopyFcn=set_param(gcbh,'PreDeleteFcn','')  PreDeleteFcn=Stateflow.SLINSF.SimulinkMan.unsafePredeleteFcn
  Double To Int8 : DataTypeConversion  OutDataTypeMode=int8  OutDataType=fixdt(1, 16)  OutScaling=2^0  OutDataTypeStr=int8  SaturateOnIntegerOverflow=on
  Embedded MATLAB Function : Stateflow chart  TreatAsAtomicUnit=on
  Gain : Gain  Gain=-1  ParameterDataType=fixdt(1, 16)  ParameterScaling=2^0  OutDataType=fixdt(1, 16)  OutScaling=2^0
  PID Controller Relative Heading : Subsystem  Description=PID
  Strafe : Outport
  wires:
  HeadingAlong/1 -> PID Controller Relative Heading/1(e), Embedded MATLAB Function/1(HeadingAlong)
  Double To Int8/1 -> Gain/1
  PID Controller Relative Heading/1(u) -> Embedded MATLAB Function/2(PIDoutput)
  Embedded MATLAB Function/1(Strafe) -> Double To Int8/1
  Gain/1 -> Strafe/1

== system brain/StateFlow Functions/StateFlowFunctions.FollowOnePath.OnePath.AlignWithPath.GetHeadings ==
  BW : Inport  PortDimensions=[120 160]  DataType=double  OutDataTypeStr=double
  f : TriggerPort  TriggerType=function-call
      settings: CopyFcn=set_param(gcbh,'PreDeleteFcn','')  PreDeleteFcn=Stateflow.SLINSF.SimulinkMan.unsafePredeleteFcn
  Display : Display
  Draw Shapes : viptextngfix/Draw Shapes  DialogController=vipDDGCreate  DialogControllerArgs=DataTag18  shape=Lines  fill=off  fillClrSource=Specify via dialog  display=User-specified value  intensity=200  color=.75  opacity=0.6  viewport=Entire image  antialiasing=off  inType=Obsolete  imagePorts=One multidimensional signal  prodOutputMode=Binary point scaling  prodOutputWordLength=32  prodOutputFracLength=14  memoryMode=Specify word length  memoryWordLength=16  memoryFracLength=15  roundingMode=Floor  overflowMode=off
  GetHeadingToPath : Stateflow chart  TreatAsAtomicUnit=on
  Hough Lines : viptransforms/Hough Lines  DialogController=vipDDGCreate  DialogControllerArgs=DataTag19  sineCompMethod=Trigonometric function  thetaRes=pi/180  firstCoeffMode=Specify word length  firstCoeffWordLength=16  firstCoeffFracLength=15  prodOutputMode=Binary point scaling  prodOutputWordLength=32  prodOutputFracLength=16  roundingMode=Nearest  overflowMode=on
  Hough Transform Stuff : Subsystem
  Image Data Type Conversion : vipconversions/Image Data Type Conversion  outDT=boolean  isSigned=on  wordLen=16  numFracBits=0
  HeadingAlongPath1 : Outport  OutDataType=fixdt(1, 16)  OutScaling=2^0
  BWout1 : Outport  Port=2  PortDimensions=[120 160]  OutDataType=fixdt(1, 16)  OutScaling=2^0
  wires:
  BW/1 -> Hough Lines/3, Draw Shapes/1, Image Data Type Conversion/1
  GetHeadingToPath/1(AlongPathHeading) -> HeadingAlongPath1/1, Display/1
  Hough Transform Stuff/1(Theta) -> GetHeadingToPath/1(Theta), Hough Lines/1
  Hough Transform Stuff/2(Rho) -> GetHeadingToPath/2(Rho), Hough Lines/2
  Hough Transform Stuff/3(Votes) -> GetHeadingToPath/3(Votes)
  Hough Lines/1 -> Draw Shapes/2
  Draw Shapes/1 -> BWout1/1
  Image Data Type Conversion/1 -> Hough Transform Stuff/1(BW)

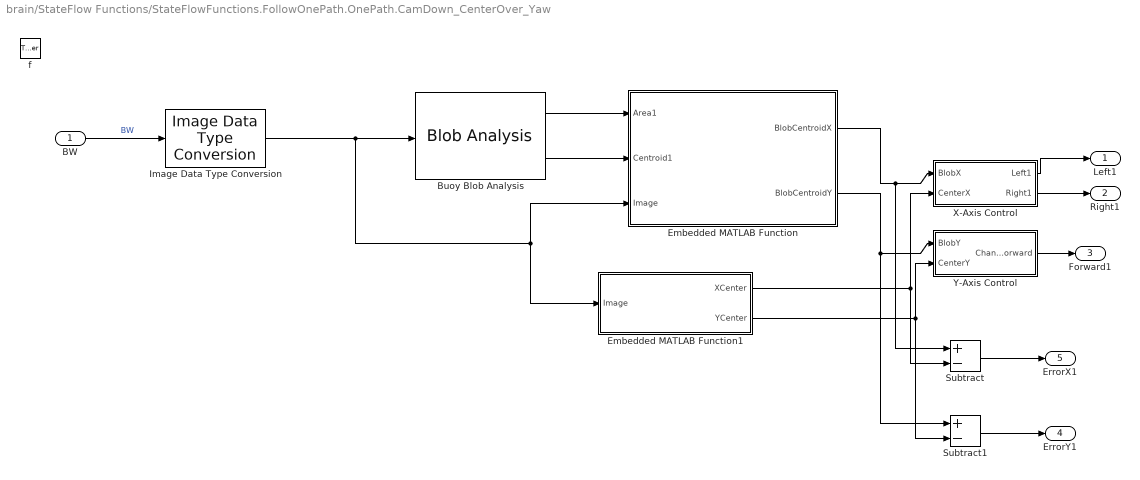
== system brain/StateFlow Functions/StateFlowFunctions.FollowOnePath.OnePath.CamDown_CenterOver_Yaw ==
  BW : Inport  PortDimensions=[120 160]
  f : TriggerPort  TriggerType=function-call
      settings: CopyFcn=set_param(gcbh,'PreDeleteFcn','')  PreDeleteFcn=Stateflow.SLINSF.SimulinkMan.unsafePredeleteFcn
  Buoy Blob Analysis : vipstatistics/Blob Analysis  Tag=vipblks_row_conv  DialogController=vipDDGCreate  DialogControllerArgs=DataTag21  area=on  centroid=on  bBox=off  majorAxis=off  minorAxis=off  angle=off  eccentricity=off  equivDiameterSq=off  extent=off  perimeter=off  maxBlobs=Max_Num_Blobs_Buoy  warnIfNumBlobsExceeded=off  isCount=off  useMinArea=on  minArea=Min_Blob_Size  useMaxArea=on  maxArea=Max_Blob_Size  excludeBorderBlob=off  outDT=double  isOutVarDim=off  isFill=on  fillValues=-1  conn=8  isLabel=off  outputMode=Binary point scaling  outputWordLength=32  outputFracLength=16  firstCoeffMode=Binary point scaling  firstCoeffWordLength=16  firstCoeffFracLength=14  secondCoeffMode=Binary point scaling  secondCoeffWordLength=32  secondCoeffFracLength=16  accumMode=Binary point scaling  accumWordLength=32  accumFracLength=0  prodOutputMode=Binary point scaling  prodOutputWordLength=32  prodOutputFracLength=16  roundingMode=Floor  overflowMode=off
  Embedded MATLAB Function : Stateflow chart  TreatAsAtomicUnit=on
  Embedded MATLAB Function1 : Stateflow chart  TreatAsAtomicUnit=on
  Image Data Type Conversion : vipconversions/Image Data Type Conversion  outDT=boolean  isSigned=on  wordLen=16  numFracBits=0
  Subtract : Sum  Inputs=+-  OutDataType=fixdt(1, 16)  OutScaling=2^-10
  Subtract1 : Sum  Inputs=+-  OutDataType=fixdt(1, 16)  OutScaling=2^-10
  X-Axis Control : Subsystem
  Y-Axis Control : Subsystem
  Left1 : Outport  OutDataType=fixdt(1, 16)  OutScaling=2^0
  Right1 : Outport  Port=2  OutDataType=fixdt(1, 16)  OutScaling=2^0
  Forward1 : Outport  Port=3  OutDataType=fixdt(1, 16)  OutScaling=2^0
  ErrorY1 : Outport  Port=4
  ErrorX1 : Outport  Port=5
  wires:
  Buoy Blob Analysis/1 -> Embedded MATLAB Function/1(Area1)
  Buoy Blob Analysis/2 -> Embedded MATLAB Function/2(Centroid1)
  Embedded MATLAB Function/1(BlobCentroidX) -> X-Axis Control/1(BlobX), Subtract/1
  Embedded MATLAB Function/2(BlobCentroidY) -> Y-Axis Control/1(BlobY), Subtract1/1
  BW/1 -> Image Data Type Conversion/1  "BW"
  Embedded MATLAB Function1/1(XCenter) -> X-Axis Control/2(CenterX), Subtract/2
  Embedded MATLAB Function1/2(YCenter) -> Y-Axis Control/2(CenterY), Subtract1/2
  X-Axis Control/1(Left1) -> Left1/1
  Y-Axis Control/1(ChangetoForward) -> Forward1/1
  Subtract/1 -> ErrorX1/1
  Subtract1/1 -> ErrorY1/1
  X-Axis Control/2(Right1) -> Right1/1
  Image Data Type Conversion/1 -> Buoy Blob Analysis/1, Embedded MATLAB Function/3(Image), Embedded MATLAB Function1/1(Image)

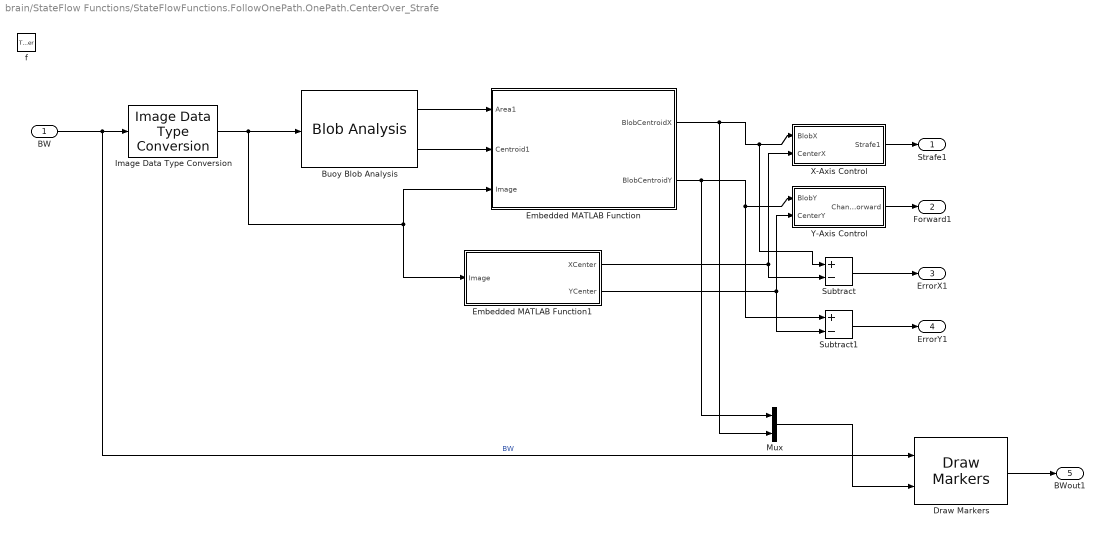
== system brain/StateFlow Functions/StateFlowFunctions.FollowOnePath.OnePath.CenterOver_Strafe ==
  BW : Inport  PortDimensions=[120 160]
  f : TriggerPort  TriggerType=function-call
      settings: CopyFcn=set_param(gcbh,'PreDeleteFcn','')  PreDeleteFcn=Stateflow.SLINSF.SimulinkMan.unsafePredeleteFcn
  Buoy Blob Analysis : vipstatistics/Blob Analysis  Tag=vipblks_row_conv  DialogController=vipDDGCreate  DialogControllerArgs=DataTag22  area=on  centroid=on  bBox=off  majorAxis=off  minorAxis=off  angle=off  eccentricity=off  equivDiameterSq=off  extent=off  perimeter=off  maxBlobs=Max_Num_Blobs_Buoy  warnIfNumBlobsExceeded=off  isCount=off  useMinArea=on  minArea=Min_Blob_Size  useMaxArea=on  maxArea=Max_Blob_Size  excludeBorderBlob=off  outDT=double  isOutVarDim=off  isFill=on  fillValues=-1  conn=8  isLabel=off  outputMode=Binary point scaling  outputWordLength=32  outputFracLength=16  firstCoeffMode=Binary point scaling  firstCoeffWordLength=16  firstCoeffFracLength=14  secondCoeffMode=Binary point scaling  secondCoeffWordLength=32  secondCoeffFracLength=16  accumMode=Binary point scaling  accumWordLength=32  accumFracLength=0  prodOutputMode=Binary point scaling  prodOutputWordLength=32  prodOutputFracLength=16  roundingMode=Floor  overflowMode=off
  Draw Markers : viptextngfix/Draw Markers  DialogController=vipDDGCreate  DialogControllerArgs=DataTag23  shape=X-mark  size=7  fill=off  fillClrSource=Specify via dialog  display=User-specified value  intensity=200  color=0.75  opacity=0.6  viewport=Entire image  antialiasing=off  inType=Obsolete  imagePorts=One multidimensional signal  prodOutputMode=Binary point scaling  prodOutputWordLength=32  prodOutputFracLength=14  memoryMode=Specify word length  memoryWordLength=16  memoryFracLength=15  roundingMode=Floor  overflowMode=off
  Embedded MATLAB Function : Stateflow chart  TreatAsAtomicUnit=on
  Embedded MATLAB Function1 : Stateflow chart  TreatAsAtomicUnit=on
  Image Data Type Conversion : vipconversions/Image Data Type Conversion  outDT=boolean  isSigned=on  wordLen=16  numFracBits=0
  Mux : Mux  Inputs=2
  Subtract : Sum  Inputs=+-  OutDataType=fixdt(1, 16)  OutScaling=2^-10
  Subtract1 : Sum  Inputs=+-  OutDataType=fixdt(1, 16)  OutScaling=2^-10
  X-Axis Control : Subsystem
  Y-Axis Control : Subsystem
  Strafe1 : Outport  OutDataType=fixdt(1, 16)  OutScaling=2^0
  Forward1 : Outport  Port=2  OutDataType=fixdt(1, 16)  OutScaling=2^0
  ErrorX1 : Outport  Port=3
  ErrorY1 : Outport  Port=4
  BWout1 : Outport  Port=5  PortDimensions=[120 160]
  wires:
  Buoy Blob Analysis/1 -> Embedded MATLAB Function/1(Area1)
  Buoy Blob Analysis/2 -> Embedded MATLAB Function/2(Centroid1)
  Embedded MATLAB Function/1(BlobCentroidX) -> X-Axis Control/1(BlobX), Subtract/1, Mux/2
  Embedded MATLAB Function/2(BlobCentroidY) -> Y-Axis Control/1(BlobY), Subtract1/1, Mux/1
  BW/1 -> Image Data Type Conversion/1, Draw Markers/1  "BW"
  Embedded MATLAB Function1/1(XCenter) -> X-Axis Control/2(CenterX), Subtract/2
  Embedded MATLAB Function1/2(YCenter) -> Y-Axis Control/2(CenterY), Subtract1/2
  X-Axis Control/1(Strafe1) -> Strafe1/1
  Y-Axis Control/1(ChangetoForward) -> Forward1/1
  Subtract/1 -> ErrorX1/1
  Subtract1/1 -> ErrorY1/1
  Image Data Type Conversion/1 -> Buoy Blob Analysis/1, Embedded MATLAB Function/3(Image), Embedded MATLAB Function1/1(Image)
  Mux/1 -> Draw Markers/2
  Draw Markers/1 -> BWout1/1

== system brain/StateFlow Functions/StateFlowFunctions.FollowOnePath.OnePath.HSVSegmentation ==
  H : Inport  PortDimensions=[120 160]  OutDataType=fixdt(1, 16)  OutScaling=2^0
  S : Inport  Port=2  PortDimensions=[120 160]  OutDataType=fixdt(1, 16)  OutScaling=2^0
  f : TriggerPort  TriggerType=function-call
      settings: CopyFcn=set_param(gcbh,'PreDeleteFcn','')  PreDeleteFcn=Stateflow.SLINSF.SimulinkMan.unsafePredeleteFcn
  Segmentation : Subsystem
  BW1 : Outport  OutDataType=fixdt(1, 16)  OutScaling=2^0
  wires:
  H/1 -> Segmentation/1(H)
  Segmentation/1(BW) -> BW1/1
  S/1 -> Segmentation/2(S)

== system brain/StateFlow Functions/StateFlowFunctions.FollowOnePath.RecognizePath.LookforTrack ==
  H : Inport  PortDimensions=[120 160]  OutDataType=fixdt(1, 16)  OutScaling=2^0
  S : Inport  Port=2  PortDimensions=[120 160]  OutDataType=fixdt(1, 16)  OutScaling=2^0
  f : TriggerPort  TriggerType=function-call
      settings: CopyFcn=set_param(gcbh,'PreDeleteFcn','')  PreDeleteFcn=Stateflow.SLINSF.SimulinkMan.unsafePredeleteFcn
  LookforTrack : Subsystem
  Image : Outport  OutDataType=fixdt(1, 16)  OutScaling=2^0
  BWout1 : Outport  Port=2  OutDataType=fixdt(1, 16)  OutScaling=2^0
  wires:
  H/1 -> LookforTrack/1(H)
  S/1 -> LookforTrack/2(S)
  LookforTrack/1(BWout) -> BWout1/1
  LookforTrack/2(Image) -> Image/1

== system brain/StateFlow Functions/StateFlowFunctions.GetDesiredDepth ==
  f : TriggerPort  TriggerType=function-call
      settings: CopyFcn=set_param(gcbh,'PreDeleteFcn','')  PreDeleteFcn=Stateflow.SLINSF.SimulinkMan.unsafePredeleteFcn
  Constant : Constant  Value=Track_Desired_Depth  OutDataType=fixdt(1, 16)  OutScaling=2^0  SampleTime=-1
  DesiredDepth : Outport
  wires:
  Constant/1 -> DesiredDepth/1
